simulink model "DC_Motor_Control_GA"  (R2021b)
settings: Solver=VariableStepAuto  StartTime=0.0  StopTime=0.2  RelTol=1e-3
model workspace (MAT data in the model file):
  J = 3.2284e-06
  Kd = 0.01
  Ke = 0.0274
  Kt = 0.0274
  L = 2.75e-06
  R = 4
  b = 3.5077e-06
libraries: slpidlib x1
settings Model: Creator=dmc-stdtest  LastModifiedBy=aulwasay
settings SolverCC: AlgebraicLoopSolver=TrustRegion
settings DataIOCC: ReturnWorkspaceOutputs=off
settings DebuggingCC: SFMachineParentedDataDiag=warning

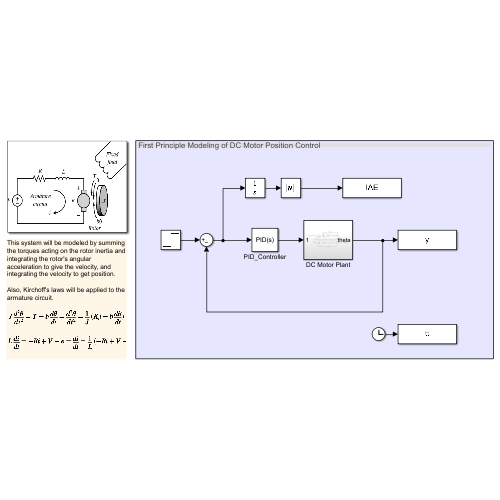
[thumbnail: Simulink's stored preview of the top-level diagram]
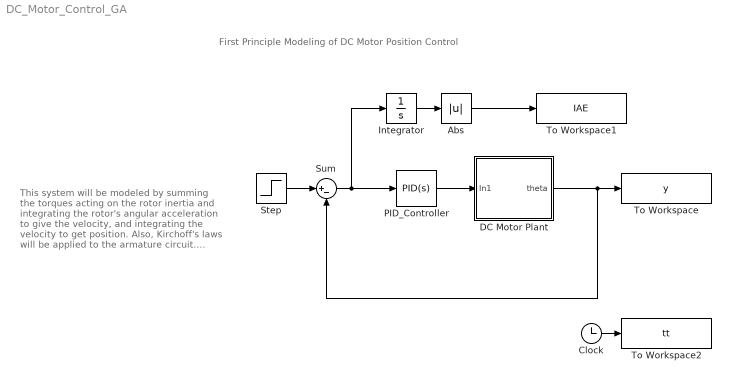
== system DC_Motor_Control_GA ==
  note: First Principle Modeling of DC Motor Position Control
  note: This system will be modeled by summing the torques acting on the rotor inertia and integrating the rotor's angular acceleration to give the velocity, and integrating the velocity to get position.
      | Also, Kirchoff's laws will be applied to the armature circuit.
      | $J\frac{d^2 \theta}{dt^2} = T - b\frac{d\theta}{dt} = \frac{d^2 \theta}{dt^2} = \frac{1}{J}(K_t i - b\frac{d\theta}{dt})$
      | $L\frac{di}{dt} = -Ri +V - e = \frac{di}{dt} = \frac{1}{L} (-Ri +V-K_b \frac{d\theta}{dt})$
  Abs : Abs
  Clock : Clock
  DC Motor Plant : Subsystem
  Integrator : Integrator
  PID_Controller : slpidlib/PID Controller  Controller=PID  Form=Parallel  TimeDomain=Continuous-time  UseExternalTs=off  SampleTime=-1  IntegratorMethod=Forward Euler  FilterMethod=Forward Euler  ControllerParametersSource=internal  P=14.6341  I=0.23964  D=0.34593  UseFilter=on  N=100  TunerSelectOption=Transfer Function Based (PID Tuner App)  InitialConditionSource=internal  InitialConditionForIntegrator=0  InitialConditionForFilter=0  DifferentiatorICPrevScaledInput=0  ExternalReset=none  TrackingMode=off  Kt=1  LimitOutput=off  SatLimitsSource=internal  UpperSaturationLimit=inf  LowerSaturationLimit=-inf  LinearizeAsGain=on  AntiWindupMode=none  Kb=1  POutMin=[]  POutMax=[]  IOutMin=[]  IOutMax=[]  DOutMin=[]  DOutMax=[]  NOutMin=[]  NOutMax=[]  SumOutMin=[]  SumOutMax=[]  SaturationOutMin=[]  SaturationOutMax=[]  PParamMin=[]  PParamMax=[]  IParamMin=[]  IParamMax=[]  DParamMin=[]  DParamMax=[]  NParamMin=[]  NParamMax=[]  KbParamMin=[]  KbParamMax=[]  KtParamMin=[]  KtParamMax=[]  KbOutMin=[]  KbOutMax=[]  KtOutMin=[]  KtOutMax=[]  IntegratorOutMin=[]  IntegratorOutMax=[]  FilterOutMin=[]  FilterOutMax=[]  SumI1OutMin=[]  SumI1OutMax=[]  SumI2OutMin=[]  SumI2OutMax=[]  SumI3OutMin=[]  SumI3OutMax=[]  SumI4OutMin=[]  SumI4OutMax=[]  SumDOutMin=[]  SumDOutMax=[]  DifferentiatorOutMin=[]  DifferentiatorOutMax=[]  FilterDiffOutCoefMin=[]  FilterDiffOutCoefMax=[]  ReciprocalOutMin=[]  ReciprocalOutMax=[]  SumDenOutMin=[]  SumDenOutMax=[]  SumNumOutMin=[]  SumNumOutMax=[]  DivideOutMin=[]  DivideOutMax=[]  UdiffTsProdOutMin=[]  UdiffTsProdOutMax=[]  NTsProdOutMin=[]  NTsProdOutMax=[]  UintegralTsProdOutMin=[]  UintegralTsProdOutMax=[]  UngainTsProdOutMin=[]  UngainTsProdOutMax=[]  IntegratorContinuousStateAttributes=''  IntegratorStateMustResolveToSignalObject=off  IntegratorRTWStateStorageClass=Auto  FilterContinuousStateAttributes=''  FilterStateMustResolveToSignalObject=off  FilterRTWStateStorageClass=Auto  ParallelPVariant=InternalParameters  IdealPVariant=Disabled  IVariant=InternalParameters  DVariant=InternalParameters  IntegratorVariant=Continuous  SatVariant=Disabled  AWVariant=Passthrough  PCopyVariant=Disabled  TRVariant=Disabled  FdbkBlocksVariant=Forward  IdealPFdbkVariant=Disabled  SatFdbkVariant=Disabled  DerivativeFilterVariant=ContFilter  NVariant=InternalParameters  NCopyVariant=Disabled  FilterICVariant=InternalICsFilter  IntegratorICVariant=InternalICs  ExternalResetVariant=Disabled  TRSumVariant=Passthrough  SumFdbkVariant=Disabled  SumVariant=Sum_PID  TsampFilterVariant=InternalTs  TsampNgainVariant=Passthrough  TsampIntegralVariant=Passthrough  ExternalSaturationOutDataTypeStr=Inherit: Same as second input
  Step : Step  Time=0  SampleTime=0.01
  Sum : Sum  Inputs=|+-
  To Workspace : ToWorkspace  VariableName=y  SampleTime=-1
  To Workspace1 : ToWorkspace  VariableName=IAE  SampleTime=-1
  To Workspace2 : ToWorkspace  VariableName=tt  SampleTime=-1
  wires:
  Step/1 -> Sum/1
  Sum/1 -> Integrator/1, PID_Controller/1
  DC Motor Plant/1(theta) -> To Workspace/1, Sum/2
  PID_Controller/1 -> DC Motor Plant/1(In1)
  Integrator/1 -> Abs/1
  Abs/1 -> To Workspace1/1
  Clock/1 -> To Workspace2/1

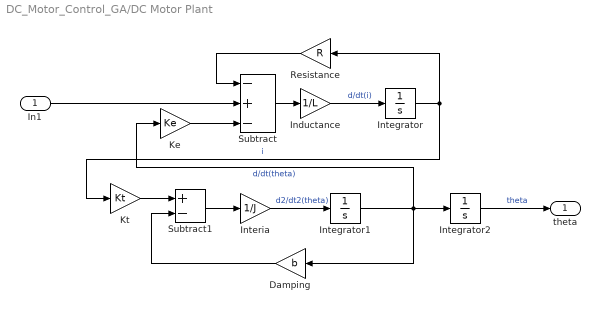
== system DC_Motor_Control_GA/DC Motor Plant ==
  In1 : Inport
  Damping : Gain  Gain=b
  Inductance : Gain  Gain=1/L
  Integrator : Integrator
  Integrator1 : Integrator
  Integrator2 : Integrator
  Interia : Gain  Gain=1/J
  Ke : Gain  Gain=Ke
  Kt : Gain  Gain=Kt
  Resistance : Gain  Gain=R
  Subtract : Sum  Inputs=-+-
  Subtract1 : Sum  Inputs=+-
  theta : Outport
  wires:
  Kt/1 -> Subtract1/1
  Inductance/1 -> Integrator/1  "d/dt(i)"
  Interia/1 -> Integrator1/1  "d2/dt2(theta)"
  Integrator/1 -> Resistance/1, Kt/1  "i"
  Subtract1/1 -> Interia/1
  Integrator1/1 -> Damping/1, Ke/1, Integrator2/1  "d/dt(theta)"
  Resistance/1 -> Subtract/1
  Damping/1 -> Subtract1/2
  Ke/1 -> Subtract/3
  Subtract/1 -> Inductance/1
  In1/1 -> Subtract/2
  Integrator2/1 -> theta/1  "theta"
